simulink model "TFlex_ISSGP_Twin"  (R2018b)
settings: Solver=VariableStepAuto  StartTime=0.0  StopTime=t_end  RelTol=1e-3
values from neighbouring files (symbols this model uses):
  beta_init = 1    [TFlex_ISSGP_Twin_init.m]    (also in TFlex_ISSGP_init.m)
  beta_min = 0.0000    (= 0)    [TFlex_ISSGP_Twin_init.m]    (also in TFlex_ISSGP_init.m)
  beta_reduc = 0.991    [TFlex_ISSGP_Twin_init.m]    (also in TFlex_ISSGP_init.m = nthroot(beta_T/beta_init,(t_hypUpdate(2)-t_hypUpdate(1))/ts_)
  bufferResamp = 50    [TFlex_ISSGP_Twin_init.m]    (also in TFlex_ISSGP_init.m = 10)
  bufferSize = 25    [TFlex_ISSGP_Twin_init.m]    (also in TFlex_ISSGP_init.m = 250)
  D = 80    [TFlex_ISSGP_Twin_init.m]    (also in TFlex_ISSGP_init.m)
  ell = ones(1,n).*0.1    [TFlex_ISSGP_Twin_init.m]    (also in TFlex_ISSGP_init.m = [0.5091   0.0036538   0.0012249])
  ell_init = ell    [TFlex_ISSGP_Twin_init.m]    (also in TFlex_ISSGP_init.m)
  mu_X = [0,0,0]    [TFlex_ISSGP_Twin_init.m]    (also in TFlex_ISSGP_init.m)
  mu_Y = 0    [TFlex_ISSGP_Twin_init.m]    (also in TFlex_ISSGP_init.m)
  n = 3    [TFlex_ISSGP_Twin_init.m]    (also in TFlex_ISSGP_init.m)
  RAND = randn(D,n)    [TFlex_ISSGP_Twin_init.m]    (also in TFlex_ISSGP_init.m)
  RAND2 = randn(D,n)    [TFlex_ISSGP_Twin_init.m]
  sf = 1    [TFlex_ISSGP_Twin_init.m]    (also in TFlex_ISSGP_init.m = 111.9926)
  sf_init = sf    (= 1)    [TFlex_ISSGP_Twin_init.m]    (also in TFlex_ISSGP_init.m = 111.9926)
  sig_X = [1,1,1]    [TFlex_ISSGP_Twin_init.m]    (also in TFlex_ISSGP_init.m)
  sig_Y = 1    [TFlex_ISSGP_Twin_init.m]    (also in TFlex_ISSGP_init.m)
  SIGMA2_init = RAND2.*ell    [TFlex_ISSGP_Twin_init.m]
  SIGMA_init = RAND.*ell    [TFlex_ISSGP_Twin_init.m]    (also in TFlex_ISSGP_init.m)
  sn = 2.303584    [TFlex_ISSGP_Twin_init.m]    (also in TFlex_ISSGP_init.m)
  sn2 = sn    (= 2.303584)    [TFlex_ISSGP_Twin_init.m]
  t_hypUpdate = [10 55]    [TFlex_ISSGP_Twin_init.m]    (also in TFlex_ISSGP_init.m = [t_end t_end+1])
  t_hypUpdate2 = [70 115]    [TFlex_ISSGP_Twin_init.m]
  t_learn = 55    [TFlex_ISSGP_Twin_init.m]    (also in TFlex_ISSGP_init.m = 5)
  t_learn2 = 115    [TFlex_ISSGP_Twin_init.m]
  t_predict = 65    [TFlex_ISSGP_Twin_init.m]    (also in TFlex_ISSGP_init.m = 15)
  t_predict2 = 125    [TFlex_ISSGP_Twin_init.m]
  ts = 1/1000    (= 0.001)    [TFlex_ISSGP_Twin_init.m]    (also in TFlex_ISSGP_init.m)
  ts_opti = ts*100    (= 0.1)    [TFlex_ISSGP_Twin_init.m]    (also in TFlex_ISSGP_init.m)
  Z = bufferSize*bufferResamp    (= 1250)    [TFlex_ISSGP_Twin_init.m]    (also in TFlex_ISSGP_init.m = 2500)
undefined symbols (not defined in the file or in its folder): Cogging, DiscIntNeverNeededParam, I_limit, PID, Plant, R1, R2, Reference, SVF, X, Y
libraries: simulink x6
settings Model: Creator=wout7  LastModifiedBy=wout7

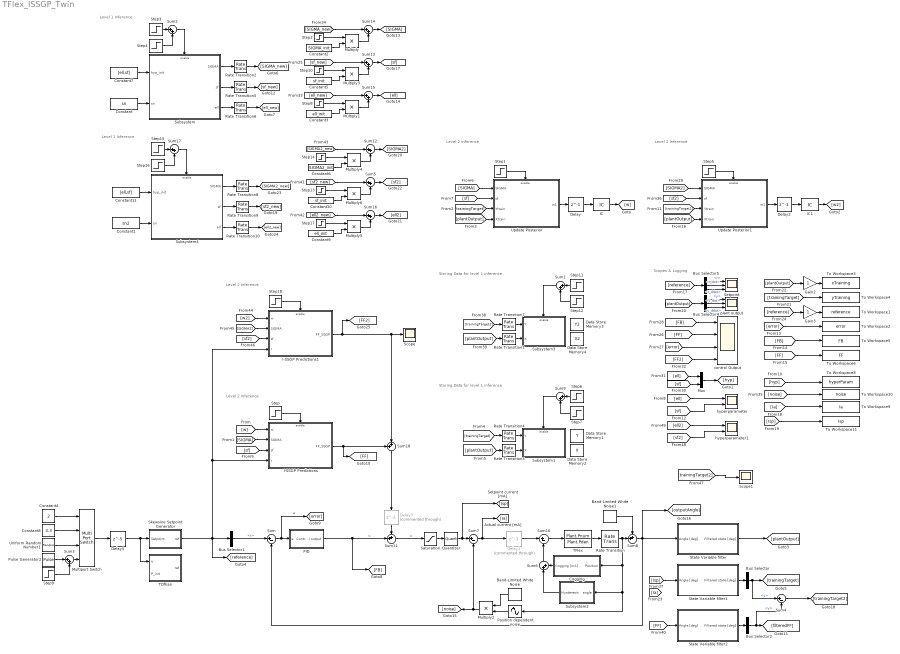
== system TFlex_ISSGP_Twin ==
  note: Storing Data for level 1 inference
  note: Scopes & Logging
  note: Level 1 Inference
  note: Level 2 Inference
  note: Level 2 Inference
  note: Level 2 Inference
  note: Storing Data for level 1 inference
  note: Level 1 Inference
  note: Level 2 Inference
  Band-Limited White Noise : simulink/Sources/Band-Limited White Noise  Cov=[1e-9]  Ts=ts  seed=48124
  Band-Limited White Noise1 : simulink/Sources/Band-Limited White Noise  Cov=[1e-15]  Ts=ts  seed=[23341]
  Bus Selector : BusSelector  OutputSignals=y
  Bus Selector1 : BusSelector  OutputSignals=r
  Bus Selector2 : BusSelector  OutputSignals=y
  Bus Selector4 : BusSelector  OutputSignals=y,y_dot,y_ddot
  Bus Selector5 : BusSelector  OutputSignals=r,r_dot,r_ddot
  Cogging : Subsystem
  Constant : Constant  Value=sn  SampleTime=ts_opti
  Constant1 : Constant  Value=sn2  SampleTime=ts_opti
  Constant10 : Constant  Value=sf_init  SampleTime=ts_opti
  Constant11 : Constant  Value=[ell,sf]  VectorParams1D=off  SampleTime=ts_opti
  Constant2 : Constant  Value=SIGMA_init  SampleTime=ts_opti
  Constant3 : Constant  Value=ell_init  SampleTime=ts_opti
  Constant4 : Constant  Value=2  SampleTime=Reference.ts
  Constant5 : Constant  Value=sf_init  SampleTime=ts_opti
  Constant6 : Constant  Value=SIGMA2_init  SampleTime=ts_opti
  Constant7 : Constant  Value=[ell,sf]  VectorParams1D=off  SampleTime=ts_opti
  Constant8 : Constant  Value=3.3  SampleTime=Reference.ts
  Constant9 : Constant  Value=ell_init  SampleTime=ts_opti
  Data Store Memory1 : DataStoreMemory  DataStoreName=Y  ReadBeforeWriteMsg=warning  WriteAfterWriteMsg=warning  WriteAfterReadMsg=warning  InitialValue=zeros(bufferSize,1)  VectorParams1D=off  ShowAdditionalParam=off  OutDataTypeStr=double
      settings: LockScale=on
  Data Store Memory2 : DataStoreMemory  DataStoreName=X  ReadBeforeWriteMsg=warning  WriteAfterWriteMsg=warning  WriteAfterReadMsg=warning  InitialValue=zeros(bufferSize,3)  VectorParams1D=off  ShowAdditionalParam=off  OutDataTypeStr=double
      settings: LockScale=on
  Data Store Memory3 : DataStoreMemory  DataStoreName=Y2  ReadBeforeWriteMsg=warning  WriteAfterWriteMsg=warning  WriteAfterReadMsg=warning  InitialValue=zeros(bufferSize,1)  VectorParams1D=off  ShowAdditionalParam=off  OutDataTypeStr=double
      settings: LockScale=on
  Data Store Memory4 : DataStoreMemory  DataStoreName=X2  ReadBeforeWriteMsg=warning  WriteAfterWriteMsg=warning  WriteAfterReadMsg=warning  InitialValue=zeros(bufferSize,3)  VectorParams1D=off  ShowAdditionalParam=off  OutDataTypeStr=double
      settings: LockScale=on
  Delay : Delay  DelayLength=1  InitialCondition=0
  Delay1 : Delay  Commented=through  DelayLength=3  InitialCondition=0
  Delay2 : Delay  DelayLength=1  InitialCondition=0
  Delay3 : Delay  Commented=through  DelayLength=3  InitialCondition=0
  Delay5 : Delay  DelayLength=5  SampleTime=Reference.ts
  Gain2 : Gain
  Gain3 : Gain
  I-SSGP Predictions : Subsystem
  I-SSGP Predictions1 : Subsystem
  IC : InitialCondition  Value=ones(2*D,1)*0.001
  IC1 : InitialCondition  Value=ones(2*D,1)*0.001
  Multiply{,1..6} (7 alike) : Product
  Multiport Switch : MultiPortSwitch
  Mux : Mux  Inputs=2
  PID : Subsystem
  Position dependent noise : Sin  TimeSource=Use external signal  Amplitude=2.5  Bias=7.4979  Frequency=2*pi/13  SampleTime=0
  Pulse Generator2 : DiscretePulseGenerator  Amplitude=2*24  SampleTime=Reference.ts
  Quantizer : Quantizer  QuantizationInterval=1
  Rate Transition{,2,5..6,8..10} (7 alike) : RateTransition  OutPortSampleTime=ts
  Rate Transition1 : RateTransition  OutPortSampleTime=ts*10
  Rate Transition3 : RateTransition  OutPortSampleTime=ts*bufferResamp
  Rate Transition4 : RateTransition  OutPortSampleTime=ts*bufferResamp
  Rate Transition7 : RateTransition  OutPortSampleTime=ts*10
  Saturation : Saturate  UpperLimit=I_limit  LowerLimit=-I_limit
  Scope : Scope
  Scope1 : Scope
  Setpoint : Scope  NumInputPorts=3
  Skewsine Setpoint Generator : Subsystem
  State Variable filter : Subsystem
  State Variable filter1 : Subsystem
  State Variable filter2 : Subsystem
  Step : Step  Time=t_predict  SampleTime=ts
  Step1 : Step  Time=t_learn  SampleTime=ts
  Step{2,8,10,13..14,17} (6 alike) : Step  Time=t_hypUpdate(1)+ts  Before=1  After=0  SampleTime=ts_opti
  Step11 : Step  Time=t_hypUpdate2(2)  After=-1  SampleTime=ts_opti
  Step12 : Step  Time=t_hypUpdate2(1)-Z*ts  SampleTime=ts_opti
  Step15 : Step  Time=t_hypUpdate2(2)  After=-1  SampleTime=ts_opti
  Step16 : Step  Time=t_hypUpdate2(1)  SampleTime=ts_opti
  Step18 : Step  Time=t_predict2  SampleTime=ts
  Step3 : Step  Time=t_hypUpdate(2)  After=-1  SampleTime=ts_opti
  Step4 : Step  Time=t_hypUpdate(1)  SampleTime=ts_opti
  Step5 : Step  Time=t_learn2  SampleTime=ts
  Step6 : Step  Time=t_hypUpdate(2)  After=-1  SampleTime=ts_opti
  Step7 : Step  Time=t_hypUpdate(1)-Z*ts  SampleTime=ts_opti
  Step9 : Step  Time=0  After=-24  SampleTime=Reference.ts
  Subsystem : Subsystem
  Subsystem1 : Subsystem
  Subsystem2 : Subsystem
  Subsystem3 : Subsystem
  Subsystem4 : Subsystem
  Sum{,4,7,10} (4 alike) : Sum  Inputs=|+-
  Sum{1..3,5..6,9,12..17} (12 alike) : Sum  Inputs=|++
  Sum11 : Sum  Inputs=++|
  Sum18 : Sum  Inputs=++|
  Sum8 : Sum  Inputs=++|
  TDfhan : Subsystem
  TFlex : TransferFcn  Numerator=Plant.Pnum  Denominator=Plant.Pden  ContinuousStateAttributes='angle'
  To Workspace1 : ToWorkspace  VariableName=reference  SampleTime=-1
  To Workspace10 : ToWorkspace  VariableName=noise  SampleTime=-1
  To Workspace11 : ToWorkspace  VariableName=Isp  SampleTime=-1
  To Workspace2 : ToWorkspace  VariableName=error  SampleTime=-1
  To Workspace3 : ToWorkspace  VariableName=xTraining  SampleTime=-1
  To Workspace4 : ToWorkspace  VariableName=yTraining  SampleTime=-1
  To Workspace5 : ToWorkspace  VariableName=FB  SampleTime=-1
  To Workspace6 : ToWorkspace  VariableName=FF  SampleTime=-1
  To Workspace8 : ToWorkspace  VariableName=hyperParam  SampleTime=-1
  To Workspace9 : ToWorkspace  VariableName=Ia  SampleTime=-1
  Uniform Random Number1 : UniformRandomNumber  Minimum=-23  Maximum=23  Seed=Reference.seed  SampleTime=Reference.ts
  Update Posterior : Subsystem
  Update Posterior1 : Subsystem
  control Output : Scope  NumInputPorts=4
  hyperparameter : Scope  NumInputPorts=2
  hyperparameter1 : Scope  NumInputPorts=2
  plant output : Scope  NumInputPorts=3
  wires:
  Sum/1 -> PID/1(e), [error]  "e"
  Sum8/1 -> State Variable filter/1(Angle [deg]), [outputAngle], Sum/2
  Bus Selector1/1 -> Sum/1  "<r>"
  Update Posterior/1(w1) -> Delay/1
  Step/1 -> I-SSGP Predictions/Enable
  Step1/1 -> Update Posterior/Enable
  IC/1 -> [w]
  [w] -> I-SSGP Predictions/1(w)
  [sf] -> Update Posterior/2(sf)
  [SIGMA] -> I-SSGP Predictions/2(SIGMA)
  Delay/1 -> IC/1
  [trainingTarget] -> Update Posterior/3(Ytrain)
  [SIGMA] -> Update Posterior/1(SIGMA)
  Constant7/1 -> Subsystem/1(hyp_init)
  Step4/1 -> Sum2/2
  Step3/1 -> Sum2/1
  Sum2/1 -> Subsystem/Enable
  [sf] -> I-SSGP Predictions/3(sf)
  TFlex/1 -> Rate Transition/1
  [reference] -> Gain3/1
  Bus Selector5/2 -> Setpoint/2  "<r_dot>"
  Bus Selector5/1 -> Setpoint/1  "<r>"
  [error] -> To Workspace2/1
  Bus Selector5/3 -> Setpoint/3  "<r_ddot>"
  [FB] -> To Workspace5/1
  [plantOutput] -> Gain2/1
  Gain2/1 -> To Workspace3/1
  [plantOutput] -> Bus Selector4/1
  Gain3/1 -> To Workspace1/1
  Bus Selector4/1 -> plant output/1  "<y>"
  Bus Selector4/3 -> plant output/3  "<y_ddot>"
  [reference] -> Bus Selector5/1
  [trainingTarget] -> To Workspace4/1
  Bus Selector4/2 -> plant output/2  "<y_dot>"
  [FF] -> To Workspace6/1
  [FF] -> control Output/2
  [error] -> control Output/3
  [FB] -> control Output/1
  Step7/1 -> Sum9/2
  Sum9/1 -> Subsystem1/Enable
  Step6/1 -> Sum9/1
  Subsystem/2(sf) -> Rate Transition5/1
  Subsystem/1(SIGMA) -> Rate Transition2/1
  Subsystem/3(ell) -> Rate Transition6/1
  [ell] -> hyperparameter/1
  [hyp] -> To Workspace8/1
  [sf] -> hyperparameter/2
  [sf] -> Mux/2
  [ell] -> Mux/1
  Mux/1 -> [hyp]
  [plantOutput] -> Rate Transition3/1
  Rate Transition3/1 -> Subsystem1/2(X)
  [trainingTarget] -> Rate Transition4/1
  Rate Transition4/1 -> Subsystem1/1(Y)
  Rate Transition2/1 -> [SIGMA_new]
  Rate Transition5/1 -> [sf_new]
  Rate Transition6/1 -> [ell_new]
  [SIGMA_new] -> Sum14/1
  Step2/1 -> Multiply/1
  Constant2/1 -> Multiply/2
  Multiply/1 -> Sum14/2
  Sum14/1 -> [SIGMA]
  [plantOutput] -> Update Posterior/4(Xtrain)
  Saturation/1 -> Quantizer/1
  PID/1(Control output) -> [FB], Sum11/2  "u"
  State Variable filter/1(Filtered state [deg]) -> [plantOutput]
  Rate Transition/1 -> Sum8/2, Cogging/1(Position), Subsystem2/1(angle), Position dependent noise/1
  Sum11/1 -> Saturation/1  "u"
  Sum10/1 -> TFlex/1
  State Variable filter1/1(Filtered state [deg]) -> Bus Selector/1
  Sum7/1 -> Delay1/1, [Ia]
  Multiply2/1 -> Sum7/2, [noise]
  [sf_new] -> Sum13/1
  Step10/1 -> Multiply3/1
  Multiply3/1 -> Sum13/2
  Sum13/1 -> [sf]
  Constant5/1 -> Multiply3/2
  [ell_new] -> Sum15/1
  Step8/1 -> Multiply1/1
  Multiply1/1 -> Sum15/2
  Sum15/1 -> [ell]
  Constant3/1 -> Multiply1/2
  Cogging/1(Cogging [mA]) -> Sum6/2
  Quantizer/1 -> [Isp], Sum7/1
  I-SSGP Predictions/1(FF_SSGP) -> [FF], Sum18/1
  Delay3/1 -> Sum11/1
  Band-Limited White Noise/1 -> Multiply2/1
  Position dependent noise/1 -> Multiply2/2
  Constant/1 -> Subsystem/2(sn)
  [noise] -> To Workspace10/1
  Pulse Generator2/1 -> Sum3/1
  Sum3/1 -> Multiport Switch/4
  Step9/1 -> Sum3/2
  Constant4/1 -> Multiport Switch/1
  Uniform Random Number1/1 -> Multiport Switch/3
  Constant8/1 -> Multiport Switch/2
  [Ia] -> To Workspace9/1
  [Isp] -> To Workspace11/1
  Band-Limited White Noise1/1 -> Sum8/1
  Delay1/1 -> Sum10/1
  [Isp] -> State Variable filter1/1(Angle [deg])
  Bus Selector/1 -> Sum4/1, [trainingTarget]  "<y>"
  Sum6/1 -> Sum10/2
  Multiport Switch/1 -> Delay5/1
  Delay5/1 -> Skewsine Setpoint Generator/1(Setpoint), TDfhan/1(V)
  Subsystem2/1(Hysteresis) -> Sum6/1
  Update Posterior1/1(w1) -> Delay2/1
  [plantOutput] -> Update Posterior1/4(Xtrain)
  IC1/1 -> [w2]
  [trainingTarget2] -> Update Posterior1/3(Ytrain)
  [sf2] -> Update Posterior1/2(sf)
  Step5/1 -> Update Posterior1/Enable
  [SIGMA2] -> Update Posterior1/1(SIGMA)
  Delay2/1 -> IC1/1
  Sum1/1 -> Subsystem3/Enable
  Step11/1 -> Sum1/1
  [plantOutput] -> Rate Transition1/1
  [trainingTarget2] -> Rate Transition7/1
  Rate Transition1/1 -> Subsystem3/2(X)
  Step12/1 -> Sum1/2
  Rate Transition7/1 -> Subsystem3/1(Y)
  [FF] -> State Variable filter2/1(Angle [deg])
  State Variable filter2/1(Filtered state [deg]) -> Bus Selector2/1
  Bus Selector2/1 -> Sum4/2, [filteredFF]  "<y>"
  Sum4/1 -> [trainingTarget2]
  Sum12/1 -> [SIGMA2]
  Rate Transition9/1 -> [sf2_new]
  Sum5/1 -> [sf2]
  Constant10/1 -> Multiply6/2
  Sum16/1 -> [ell2]
  Step17/1 -> Multiply5/1
  Step13/1 -> Multiply6/1
  [ell2_new] -> Sum16/1
  Constant9/1 -> Multiply5/2
  Step15/1 -> Sum17/1
  Multiply5/1 -> Sum16/2
  Multiply6/1 -> Sum5/2
  [SIGMA2_new] -> Sum12/1
  Rate Transition10/1 -> [ell2_new]
  Rate Transition8/1 -> [SIGMA2_new]
  Constant6/1 -> Multiply4/2
  Constant1/1 -> Subsystem4/2(sn)
  Subsystem4/1(SIGMA) -> Rate Transition8/1
  Subsystem4/3(ell) -> Rate Transition10/1
  Multiply4/1 -> Sum12/2
  Constant11/1 -> Subsystem4/1(hyp_init)
  Subsystem4/2(sf) -> Rate Transition9/1
  [sf2_new] -> Sum5/1
  Sum17/1 -> Subsystem4/Enable
  Step16/1 -> Sum17/2
  Step14/1 -> Multiply4/1
  [w2] -> I-SSGP Predictions1/1(w)
  Step18/1 -> I-SSGP Predictions1/Enable
  Skewsine Setpoint Generator/1(ref) -> I-SSGP Predictions1/4(r), I-SSGP Predictions/4(r), [reference], Bus Selector1/1
  [sf2] -> I-SSGP Predictions1/3(sf)
  [SIGMA2] -> I-SSGP Predictions1/2(SIGMA)
  Sum18/1 -> Delay3/1
  I-SSGP Predictions1/1(FF_SSGP) -> [FF2], Sum18/2, Scope/1
  [trainingTarget2] -> Scope1/1
  [ell2] -> hyperparameter1/1
  [sf2] -> hyperparameter1/2
  [FF2] -> control Output/4

== system TFlex_ISSGP_Twin/Cogging ==
  Position : Inport
  Gain : Gain  Gain=20
  Scope : Scope
  Sine Wave Function : Sin  TimeSource=Use external signal  Amplitude=Cogging.amplitude  Frequency=2*pi./Cogging.frequency  Phase=Cogging.phase*2*pi  SampleTime=0
  Sum of Elements : Sum  Inputs=+
  Cogging [mA] : Outport
  wires:
  Gain/1 -> Scope/1, [Cogging], Cogging [mA]/1
  Sum of Elements/1 -> Gain/1
  Position/1 -> Sine Wave Function/1
  Sine Wave Function/1 -> Sum of Elements/1

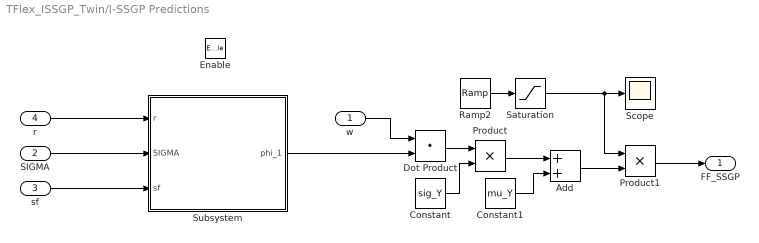
== system TFlex_ISSGP_Twin/I-SSGP Predictions ==
  w : Inport
  SIGMA : Inport  Port=2
  sf : Inport  Port=3
  r : Inport  Port=4
  Enable : EnablePort
  Add : Sum
  Constant : Constant  Value=sig_Y  VectorParams1D=off  SampleTime=ts
  Constant1 : Constant  Value=mu_Y  VectorParams1D=off  SampleTime=ts
  Dot Product : DotProduct  OutDataTypeStr=Inherit: Inherit via internal rule
  Product : Product
  Product1 : Product
  Ramp2 : simulink/Sources/Ramp  slope=1/10  start=t_predict  InitialOutput=0
  Saturation : Saturate  UpperLimit=1  LowerLimit=0
  Scope : Scope
  Subsystem : Subsystem
  FF_SSGP : Outport  SampleTime=ts
  wires:
  w/1 -> Dot Product/1
  Subsystem/1(phi_1) -> Dot Product/2
  SIGMA/1 -> Subsystem/2(SIGMA)
  Dot Product/1 -> Product/1
  Constant/1 -> Product/2
  Product/1 -> Add/1
  Constant1/1 -> Add/2
  Product1/1 -> FF_SSGP/1
  Ramp2/1 -> Saturation/1
  Add/1 -> Product1/2
  sf/1 -> Subsystem/3(sf)
  Saturation/1 -> Product1/1, Scope/1
  r/1 -> Subsystem/1(r)

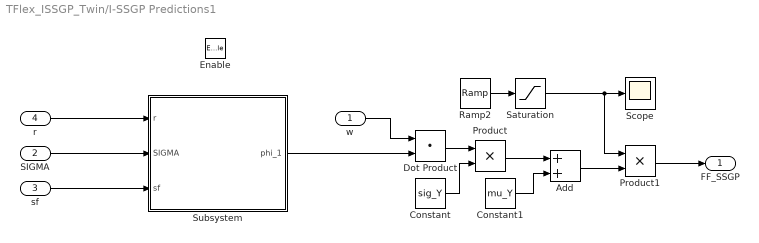
== system TFlex_ISSGP_Twin/I-SSGP Predictions1 ==
  w : Inport
  SIGMA : Inport  Port=2
  sf : Inport  Port=3
  r : Inport  Port=4
  Enable : EnablePort
  Add : Sum
  Constant : Constant  Value=sig_Y  VectorParams1D=off  SampleTime=ts
  Constant1 : Constant  Value=mu_Y  VectorParams1D=off  SampleTime=ts
  Dot Product : DotProduct  OutDataTypeStr=Inherit: Inherit via internal rule
  Product : Product
  Product1 : Product
  Ramp2 : simulink/Sources/Ramp  slope=1/10  start=t_predict  InitialOutput=0
  Saturation : Saturate  UpperLimit=1  LowerLimit=0
  Scope : Scope
  Subsystem : Subsystem
  FF_SSGP : Outport  SampleTime=ts
  wires:
  w/1 -> Dot Product/1
  Subsystem/1(phi_1) -> Dot Product/2
  SIGMA/1 -> Subsystem/2(SIGMA)
  Dot Product/1 -> Product/1
  Constant/1 -> Product/2
  Product/1 -> Add/1
  Constant1/1 -> Add/2
  Product1/1 -> FF_SSGP/1
  Ramp2/1 -> Saturation/1
  Add/1 -> Product1/2
  sf/1 -> Subsystem/3(sf)
  Saturation/1 -> Product1/1, Scope/1
  r/1 -> Subsystem/1(r)

== system TFlex_ISSGP_Twin/PID ==
  e : Inport
  Discrete Derivative : simulink/Discrete/Discrete Derivative  gainval=1.0  ICPrevScaledInput=0.0  OutMin=[]  OutMax=[]  OutDataType=fixdt(1, 16)  OutScaling=2^-10  DoSatur=off
  Discrete-Time Integrator2 : DiscreteIntegrator  SampleTime=-1  ICPrevOutput=DiscIntNeverNeededParam  ICPrevScaledInput=DiscIntNeverNeededParam
  Gain1 : Gain  Gain=PID.Kp
  Gain2 : Gain  Gain=PID.Ki
  Gain3 : Gain  Gain=PID.Kd
  Lowpass : DiscreteTransferFcn  Numerator=PID.LPnum  Denominator=PID.LPden  SampleTime=ts
  Sum2 : Sum  Inputs=3
  Control output : Outport
  wires:
  Discrete-Time Integrator2/1 -> Gain2/1
  Gain1/1 -> Sum2/2
  Gain2/1 -> Sum2/1
  Gain3/1 -> Sum2/3
  Sum2/1 -> Control output/1
  e/1 -> Discrete-Time Integrator2/1, Gain1/1, Lowpass/1
  Lowpass/1 -> Discrete Derivative/1
  Discrete Derivative/1 -> Gain3/1

== system TFlex_ISSGP_Twin/Skewsine Setpoint Generator ==
  Setpoint : Inport
  Bus Creator : BusCreator  Inputs=3
  Subsystem : Subsystem
  ref : Outport
  wires:
  Subsystem/3(r_ddot) -> Bus Creator/3  "r_ddot"
  Bus Creator/1 -> ref/1
  Subsystem/2(r_dot) -> Bus Creator/2  "r_dot"
  Subsystem/1(r) -> Bus Creator/1  "r"
  Setpoint/1 -> Subsystem/1(setpoint)

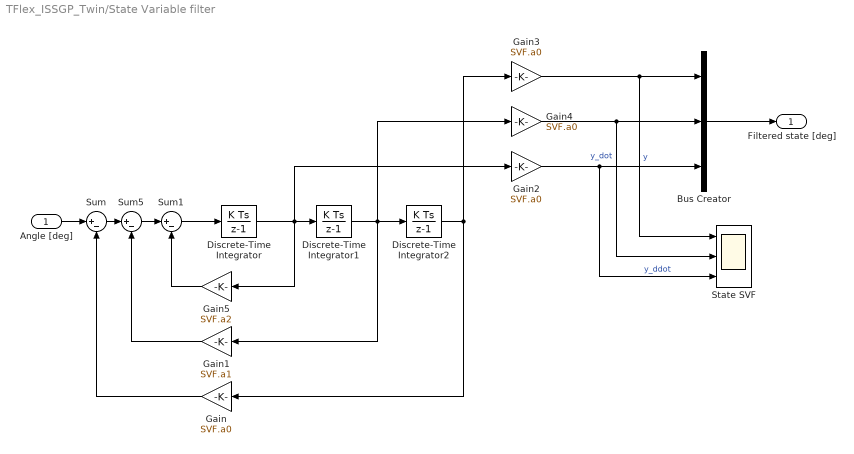
== system TFlex_ISSGP_Twin/State Variable filter ==
  Angle [deg] : Inport
  Bus Creator : BusCreator  Inputs=3
  Discrete-Time Integrator : DiscreteIntegrator  SampleTime=-1  ICPrevOutput=DiscIntNeverNeededParam  ICPrevScaledInput=DiscIntNeverNeededParam
  Discrete-Time Integrator1 : DiscreteIntegrator  SampleTime=-1  ICPrevOutput=DiscIntNeverNeededParam  ICPrevScaledInput=DiscIntNeverNeededParam
  Discrete-Time Integrator2 : DiscreteIntegrator  SampleTime=-1  ICPrevOutput=DiscIntNeverNeededParam  ICPrevScaledInput=DiscIntNeverNeededParam
  Gain{,2..4} (4 alike) : Gain  Gain=SVF.a0
  Gain1 : Gain  Gain=SVF.a1
  Gain5 : Gain  Gain=SVF.a2
  State SVF : Scope  NumInputPorts=3
  Sum : Sum  Inputs=|+-
  Sum1 : Sum  Inputs=|+-
  Sum5 : Sum  Inputs=|+-
  Filtered state [deg] : Outport  SampleTime=ts
  wires:
  Bus Creator/1 -> Filtered state [deg]/1
  Sum1/1 -> Discrete-Time Integrator/1
  Angle [deg]/1 -> Sum/1
  Sum/1 -> Sum5/1
  Gain/1 -> Sum/2
  Gain1/1 -> Sum5/2
  Gain3/1 -> State SVF/1, Bus Creator/1  "y"
  Gain2/1 -> State SVF/3, Bus Creator/3  "y_ddot"
  Gain4/1 -> State SVF/2, Bus Creator/2  "y_dot"
  Gain5/1 -> Sum1/2
  Sum5/1 -> Sum1/1
  Discrete-Time Integrator/1 -> Discrete-Time Integrator1/1, Gain2/1, Gain5/1
  Discrete-Time Integrator1/1 -> Discrete-Time Integrator2/1, Gain4/1, Gain1/1
  Discrete-Time Integrator2/1 -> Gain3/1, Gain/1

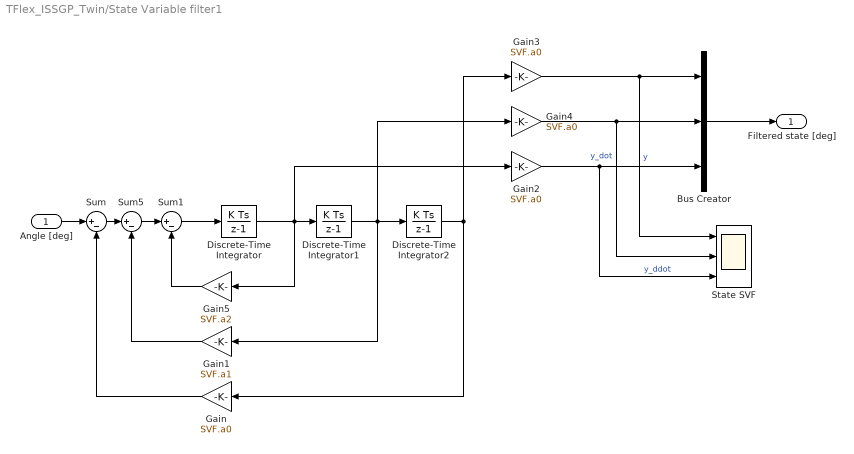
== system TFlex_ISSGP_Twin/State Variable filter1 ==
  Angle [deg] : Inport
  Bus Creator : BusCreator  Inputs=3
  Discrete-Time Integrator : DiscreteIntegrator  SampleTime=-1  ICPrevOutput=DiscIntNeverNeededParam  ICPrevScaledInput=DiscIntNeverNeededParam
  Discrete-Time Integrator1 : DiscreteIntegrator  SampleTime=-1  ICPrevOutput=DiscIntNeverNeededParam  ICPrevScaledInput=DiscIntNeverNeededParam
  Discrete-Time Integrator2 : DiscreteIntegrator  SampleTime=-1  ICPrevOutput=DiscIntNeverNeededParam  ICPrevScaledInput=DiscIntNeverNeededParam
  Gain{,2..4} (4 alike) : Gain  Gain=SVF.a0
  Gain1 : Gain  Gain=SVF.a1
  Gain5 : Gain  Gain=SVF.a2
  State SVF : Scope  NumInputPorts=3
  Sum : Sum  Inputs=|+-
  Sum1 : Sum  Inputs=|+-
  Sum5 : Sum  Inputs=|+-
  Filtered state [deg] : Outport  SampleTime=ts
  wires:
  Bus Creator/1 -> Filtered state [deg]/1
  Sum1/1 -> Discrete-Time Integrator/1
  Angle [deg]/1 -> Sum/1
  Sum/1 -> Sum5/1
  Gain/1 -> Sum/2
  Gain1/1 -> Sum5/2
  Gain3/1 -> State SVF/1, Bus Creator/1  "y"
  Gain2/1 -> State SVF/3, Bus Creator/3  "y_ddot"
  Gain4/1 -> State SVF/2, Bus Creator/2  "y_dot"
  Gain5/1 -> Sum1/2
  Sum5/1 -> Sum1/1
  Discrete-Time Integrator/1 -> Discrete-Time Integrator1/1, Gain2/1, Gain5/1
  Discrete-Time Integrator1/1 -> Discrete-Time Integrator2/1, Gain4/1, Gain1/1
  Discrete-Time Integrator2/1 -> Gain3/1, Gain/1

== system TFlex_ISSGP_Twin/State Variable filter2 ==
  Angle [deg] : Inport
  Bus Creator : BusCreator  Inputs=3
  Discrete-Time Integrator : DiscreteIntegrator  SampleTime=-1  ICPrevOutput=DiscIntNeverNeededParam  ICPrevScaledInput=DiscIntNeverNeededParam
  Discrete-Time Integrator1 : DiscreteIntegrator  SampleTime=-1  ICPrevOutput=DiscIntNeverNeededParam  ICPrevScaledInput=DiscIntNeverNeededParam
  Discrete-Time Integrator2 : DiscreteIntegrator  SampleTime=-1  ICPrevOutput=DiscIntNeverNeededParam  ICPrevScaledInput=DiscIntNeverNeededParam
  Gain{,2..4} (4 alike) : Gain  Gain=SVF.a0
  Gain1 : Gain  Gain=SVF.a1
  Gain5 : Gain  Gain=SVF.a2
  State SVF : Scope  NumInputPorts=3
  Sum : Sum  Inputs=|+-
  Sum1 : Sum  Inputs=|+-
  Sum5 : Sum  Inputs=|+-
  Filtered state [deg] : Outport  SampleTime=ts
  wires:
  Bus Creator/1 -> Filtered state [deg]/1
  Sum1/1 -> Discrete-Time Integrator/1
  Angle [deg]/1 -> Sum/1
  Sum/1 -> Sum5/1
  Gain/1 -> Sum/2
  Gain1/1 -> Sum5/2
  Gain3/1 -> State SVF/1, Bus Creator/1  "y"
  Gain2/1 -> State SVF/3, Bus Creator/3  "y_ddot"
  Gain4/1 -> State SVF/2, Bus Creator/2  "y_dot"
  Gain5/1 -> Sum1/2
  Sum5/1 -> Sum1/1
  Discrete-Time Integrator/1 -> Discrete-Time Integrator1/1, Gain2/1, Gain5/1
  Discrete-Time Integrator1/1 -> Discrete-Time Integrator2/1, Gain4/1, Gain1/1
  Discrete-Time Integrator2/1 -> Gain3/1, Gain/1

== system TFlex_ISSGP_Twin/Subsystem ==
  hyp_init : Inport  PortDimensions=[1,n+1]
  sn : Inport  Port=2
  Enable : EnablePort
  Bus Creator : BusCreator  Inputs=3
  Constant13 : Constant  Value=RAND  VectorParams1D=off  SampleTime=ts_opti
  Data Store Read : DataStoreRead  DataStoreName=Y  SampleTime=ts_opti  DataStoreElements=Y(:,:)
  Data Store Read1 : DataStoreRead  DataStoreName=X  SampleTime=ts_opti  DataStoreElements=X(:,:)
  Demux : Demux
  MATLAB Function : MATLAB Function  TreatAsAtomicUnit=on
  MATLAB Function1 : MATLAB Function  TreatAsAtomicUnit=on
  Scope : Scope
  SIGMA : Outport
  sf : Outport  Port=2
  ell : Outport  Port=3
  wires:
  hyp_init/1 -> MATLAB Function/1(hyp_init)
  MATLAB Function/2(beta_out) -> Scope/1  "beta"
  Data Store Read1/1 -> MATLAB Function/2(x)
  Data Store Read/1 -> MATLAB Function/3(y)
  sn/1 -> MATLAB Function/4(sn2)
  Demux/4 -> sf/1  "sf"
  Constant13/1 -> MATLAB Function1/1(RAND)
  MATLAB Function1/1(SIGMA) -> SIGMA/1
  MATLAB Function/1(hyp_opt) -> Demux/1, MATLAB Function1/2(hyp)
  Demux/1 -> Bus Creator/1  "l_1"
  Demux/2 -> Bus Creator/2  "l_2"
  Demux/3 -> Bus Creator/3  "l_3"
  Bus Creator/1 -> ell/1

== system TFlex_ISSGP_Twin/Subsystem1 ==
  Y : Inport
  X : Inport  Port=2
  Enable : EnablePort
  Add1 : Sum  Inputs=+-
  Add2 : Sum  Inputs=+-
  Bus Selector : BusSelector  OutputSignals=y,y_dot,y_ddot
  Constant3 : Constant  Value=sig_X  VectorParams1D=off  SampleTime=ts_opti
  Constant4 : Constant  Value=mu_X  VectorParams1D=off  SampleTime=ts_opti
  Constant8 : Constant  Value=sig_Y  VectorParams1D=off  SampleTime=ts_opti
  Constant9 : Constant  Value=mu_Y  VectorParams1D=off  SampleTime=ts_opti
  Divide : Product  Inputs=*/
  Divide1 : Product  Inputs=*/
  MATLAB Function1 : MATLAB Function  TreatAsAtomicUnit=on
  MATLAB Function2 : MATLAB Function  TreatAsAtomicUnit=on
  Scope : Scope  NumInputPorts=3
  wires:
  Divide1/1 -> MATLAB Function2/1(x)
  Y/1 -> Add1/1
  Divide/1 -> MATLAB Function1/1(y)
  Add1/1 -> Divide/1
  Add2/1 -> Divide1/1
  Constant9/1 -> Add1/2
  Constant3/1 -> Divide1/2
  Constant4/1 -> Add2/2
  Constant8/1 -> Divide/2
  Bus Selector/1 -> Scope/1  "<y>"
  Bus Selector/2 -> Scope/2  "<y_dot>"
  Bus Selector/3 -> Scope/3  "<y_ddot>"
  X/1 -> Add2/1, Bus Selector/1

== system TFlex_ISSGP_Twin/Subsystem2 ==
  angle : Inport
  Discrete Derivative : simulink/Discrete/Discrete Derivative  gainval=1.0  ICPrevScaledInput=0.0  OutMin=[]  OutMax=[]  OutDataType=fixdt(1, 16)  OutScaling=2^-10  DoSatur=off
  Discrete-Time Integrator : DiscreteIntegrator  SampleTime=-1  ICPrevOutput=DiscIntNeverNeededParam  ICPrevScaledInput=DiscIntNeverNeededParam
  MATLAB Function : MATLAB Function  TreatAsAtomicUnit=on
  Sum1 : Sum  Inputs=|+-
  Hysteresis : Outport
  wires:
  MATLAB Function/1(y) -> Sum1/2
  angle/1 -> Discrete Derivative/1
  Sum1/1 -> Discrete-Time Integrator/1
  Discrete Derivative/1 -> Sum1/1, MATLAB Function/1(Vr)
  Discrete-Time Integrator/1 -> Hysteresis/1, MATLAB Function/2(p)

== system TFlex_ISSGP_Twin/Subsystem3 ==
  Y : Inport
  X : Inport  Port=2
  Enable : EnablePort
  Add1 : Sum  Inputs=+-
  Add2 : Sum  Inputs=+-
  Bus Selector : BusSelector  OutputSignals=y,y_dot,y_ddot
  Constant3 : Constant  Value=sig_X  VectorParams1D=off  SampleTime=ts_opti
  Constant4 : Constant  Value=mu_X  VectorParams1D=off  SampleTime=ts_opti
  Constant8 : Constant  Value=sig_Y  VectorParams1D=off  SampleTime=ts_opti
  Constant9 : Constant  Value=mu_Y  VectorParams1D=off  SampleTime=ts_opti
  Divide : Product  Inputs=*/
  Divide1 : Product  Inputs=*/
  MATLAB Function1 : MATLAB Function  TreatAsAtomicUnit=on
  MATLAB Function2 : MATLAB Function  TreatAsAtomicUnit=on
  Scope : Scope  NumInputPorts=4
  wires:
  Divide1/1 -> MATLAB Function2/1(x)
  Y/1 -> Scope/1, Add1/1
  Divide/1 -> MATLAB Function1/1(y)
  Add1/1 -> Divide/1
  Add2/1 -> Divide1/1
  Constant9/1 -> Add1/2
  Constant3/1 -> Divide1/2
  Constant4/1 -> Add2/2
  Constant8/1 -> Divide/2
  Bus Selector/1 -> Scope/2  "<y>"
  Bus Selector/2 -> Scope/3  "<y_dot>"
  Bus Selector/3 -> Scope/4  "<y_ddot>"
  X/1 -> Add2/1, Bus Selector/1

== system TFlex_ISSGP_Twin/Subsystem4 ==
  hyp_init : Inport  PortDimensions=[1,n+1]
  sn : Inport  Port=2
  Enable : EnablePort
  Bus Creator : BusCreator  Inputs=3
  Constant13 : Constant  Value=RAND2  VectorParams1D=off  SampleTime=ts_opti
  Data Store Read : DataStoreRead  DataStoreName=Y2  SampleTime=ts_opti  DataStoreElements=Y2
  Data Store Read1 : DataStoreRead  DataStoreName=X2  SampleTime=ts_opti  DataStoreElements=X2
  Demux : Demux
  MATLAB Function : MATLAB Function  TreatAsAtomicUnit=on
  MATLAB Function1 : MATLAB Function  TreatAsAtomicUnit=on
  Scope : Scope
  SIGMA : Outport
  sf : Outport  Port=2
  ell : Outport  Port=3
  wires:
  hyp_init/1 -> MATLAB Function/1(hyp_init)
  MATLAB Function/2(beta_out) -> Scope/1  "beta"
  Data Store Read1/1 -> MATLAB Function/2(x)
  Data Store Read/1 -> MATLAB Function/3(y)
  sn/1 -> MATLAB Function/4(sn2)
  Demux/4 -> sf/1  "sf"
  Constant13/1 -> MATLAB Function1/1(RAND)
  MATLAB Function1/1(SIGMA) -> SIGMA/1
  MATLAB Function/1(hyp_opt) -> Demux/1, MATLAB Function1/2(hyp)
  Demux/1 -> Bus Creator/1  "l_1"
  Demux/2 -> Bus Creator/2  "l_2"
  Demux/3 -> Bus Creator/3  "l_3"
  Bus Creator/1 -> ell/1

== system TFlex_ISSGP_Twin/TDfhan ==
  V : Inport
  P_init : Inport  Port=2
  Bus Creator : BusCreator  Inputs=3
  Constant : Constant  Value=Reference.transient.r  SampleTime=ts
  Constant1 : Constant  Value=Reference.transient.h  SampleTime=ts
  Discrete-Time Integrator : DiscreteIntegrator  gainval=1  SampleTime=ts  ICPrevOutput=DiscIntNeverNeededParam  ICPrevScaledInput=DiscIntNeverNeededParam
  Discrete-Time Integrator1 : DiscreteIntegrator  gainval=1  InitialConditionSource=external  InitialCondition=-24  SampleTime=ts  ICPrevOutput=DiscIntNeverNeededParam  ICPrevScaledInput=DiscIntNeverNeededParam
  MATLAB Function2 : MATLAB Function  TreatAsAtomicUnit=on
  Scope : Scope  NumInputPorts=3
  Sum : Sum  Inputs=+-|
  ref : Outport
  wires:
  Sum/1 -> MATLAB Function2/1(v1)
  V/1 -> Sum/2
  Constant/1 -> MATLAB Function2/3(r0)
  Constant1/1 -> MATLAB Function2/4(h0)
  P_init/1 -> Discrete-Time Integrator1/2
  Discrete-Time Integrator1/1 -> Sum/1, Scope/1, Bus Creator/1  "r"
  Discrete-Time Integrator/1 -> Discrete-Time Integrator1/1, Scope/2, Bus Creator/2, MATLAB Function2/2(v2)  "r_dot"
  Bus Creator/1 -> ref/1
  MATLAB Function2/1(output) -> Scope/3, Bus Creator/3, Discrete-Time Integrator/1  "r_ddot"

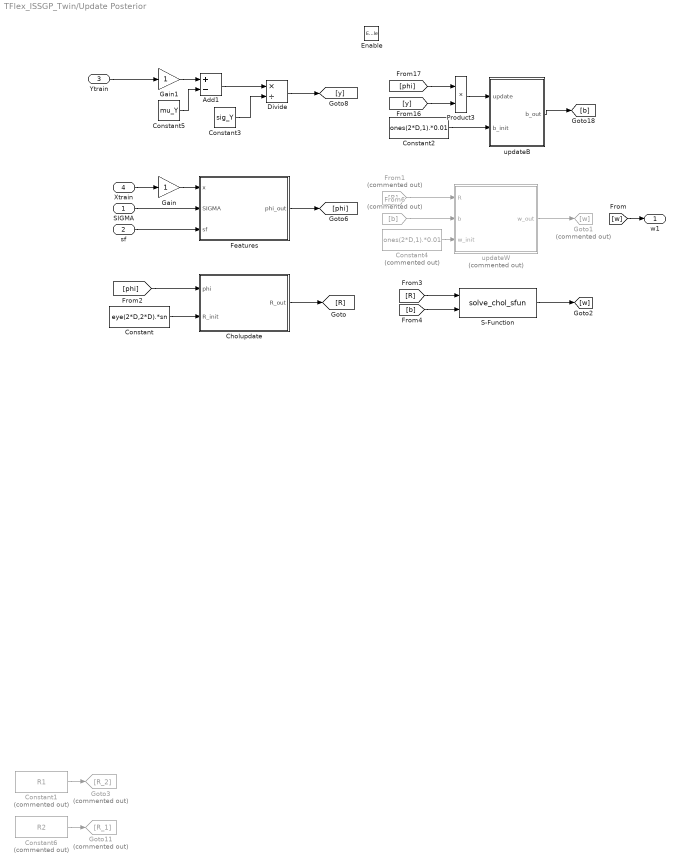
== system TFlex_ISSGP_Twin/Update Posterior ==
  SIGMA : Inport  SampleTime=ts
  sf : Inport  Port=2  SampleTime=ts
  Ytrain : Inport  Port=3  PortDimensions=[1,1]  SampleTime=ts
  Xtrain : Inport  Port=4  PortDimensions=[n,1]  SampleTime=ts
  Enable : EnablePort
  Add1 : Sum  Inputs=+-
  Cholupdate : MATLAB Function  TreatAsAtomicUnit=on
  Constant : Constant  Value=eye(2*D,2*D).*sn  SampleTime=ts
  Constant1 : Constant  Commented=on  Value=R1  VectorParams1D=off  SampleTime=-1
  Constant2 : Constant  Value=ones(2*D,1).*0.01  SampleTime=ts
  Constant3 : Constant  Value=sig_Y  VectorParams1D=off  SampleTime=ts
  Constant4 : Constant  Commented=on  Value=ones(2*D,1).*0.01  SampleTime=ts
  Constant5 : Constant  Value=mu_Y  VectorParams1D=off  SampleTime=ts
  Constant6 : Constant  Commented=on  Value=R2  VectorParams1D=off  SampleTime=-1
  Divide : Product  Inputs=*/
  Features : Subsystem
  From1 : From  Commented=on  GotoTag=R
  From6 : From  Commented=on  GotoTag=b
  Gain : Gain
  Gain1 : Gain
  Goto1 : Goto  Commented=on  GotoTag=w
  Goto11 : Goto  Commented=on  GotoTag=R_1
  Goto3 : Goto  Commented=on  GotoTag=R_2
  Product3 : Product
  S-Function : S-Function  FunctionName=solve_chol_sfun  Parameters=2*D  SFunctionDeploymentMode=off  EnableBusSupport=off
  updateB : MATLAB Function  TreatAsAtomicUnit=on
  updateW : MATLAB Function  Commented=on  TreatAsAtomicUnit=on
  w1 : Outport
  wires:
  Divide/1 -> [y]
  [phi] -> Cholupdate/1(phi)
  Features/1(phi_out) -> [phi]
  Cholupdate/1(R_out) -> [R]
  Constant3/1 -> Divide/2
  Constant5/1 -> Add1/2
  Add1/1 -> Divide/1
  From1/1 -> updateW/1(R)
  From6/1 -> updateW/2(b)
  Constant1/1 -> Goto3/1
  Constant6/1 -> Goto11/1
  [y] -> Product3/2
  [phi] -> Product3/1
  Product3/1 -> updateB/1(update)
  updateB/1(b_out) -> [b]
  SIGMA/1 -> Features/2(SIGMA)
  sf/1 -> Features/3(sf)
  Gain/1 -> Features/1(x)
  Gain1/1 -> Add1/1
  Constant/1 -> Cholupdate/2(R_init)
  Constant2/1 -> updateB/2(b_init)
  Constant4/1 -> updateW/3(w_init)
  Ytrain/1 -> Gain1/1
  Xtrain/1 -> Gain/1
  [R] -> S-Function/1
  [b] -> S-Function/2
  [w] -> w1/1
  updateW/1(w_out) -> Goto1/1
  S-Function/1 -> [w]

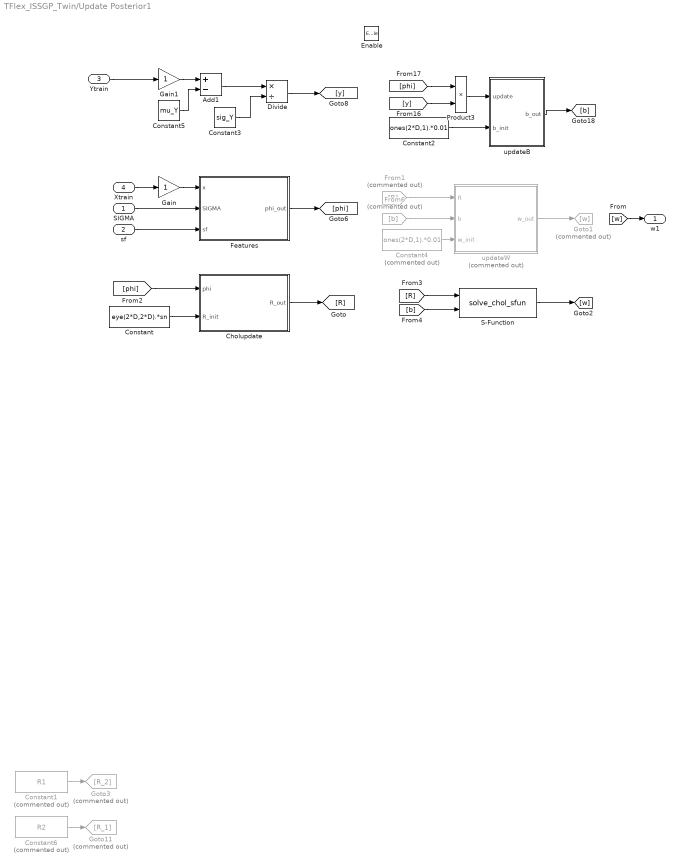
== system TFlex_ISSGP_Twin/Update Posterior1 ==
  SIGMA : Inport  SampleTime=ts
  sf : Inport  Port=2  SampleTime=ts
  Ytrain : Inport  Port=3  PortDimensions=[1,1]  SampleTime=ts
  Xtrain : Inport  Port=4  PortDimensions=[n,1]  SampleTime=ts
  Enable : EnablePort
  Add1 : Sum  Inputs=+-
  Cholupdate : MATLAB Function  TreatAsAtomicUnit=on
  Constant : Constant  Value=eye(2*D,2*D).*sn  SampleTime=ts
  Constant1 : Constant  Commented=on  Value=R1  VectorParams1D=off  SampleTime=-1
  Constant2 : Constant  Value=ones(2*D,1).*0.01  SampleTime=ts
  Constant3 : Constant  Value=sig_Y  VectorParams1D=off  SampleTime=ts
  Constant4 : Constant  Commented=on  Value=ones(2*D,1).*0.01  SampleTime=ts
  Constant5 : Constant  Value=mu_Y  VectorParams1D=off  SampleTime=ts
  Constant6 : Constant  Commented=on  Value=R2  VectorParams1D=off  SampleTime=-1
  Divide : Product  Inputs=*/
  Features : Subsystem
  From1 : From  Commented=on  GotoTag=R
  From6 : From  Commented=on  GotoTag=b
  Gain : Gain
  Gain1 : Gain
  Goto1 : Goto  Commented=on  GotoTag=w
  Goto11 : Goto  Commented=on  GotoTag=R_1
  Goto3 : Goto  Commented=on  GotoTag=R_2
  Product3 : Product
  S-Function : S-Function  FunctionName=solve_chol_sfun  Parameters=2*D  SFunctionDeploymentMode=off  EnableBusSupport=off
  updateB : MATLAB Function  TreatAsAtomicUnit=on
  updateW : MATLAB Function  Commented=on  TreatAsAtomicUnit=on
  w1 : Outport
  wires:
  Divide/1 -> [y]
  [phi] -> Cholupdate/1(phi)
  Features/1(phi_out) -> [phi]
  Cholupdate/1(R_out) -> [R]
  Constant3/1 -> Divide/2
  Constant5/1 -> Add1/2
  Add1/1 -> Divide/1
  From1/1 -> updateW/1(R)
  From6/1 -> updateW/2(b)
  Constant1/1 -> Goto3/1
  Constant6/1 -> Goto11/1
  [y] -> Product3/2
  [phi] -> Product3/1
  Product3/1 -> updateB/1(update)
  updateB/1(b_out) -> [b]
  SIGMA/1 -> Features/2(SIGMA)
  sf/1 -> Features/3(sf)
  Gain/1 -> Features/1(x)
  Gain1/1 -> Add1/1
  Constant/1 -> Cholupdate/2(R_init)
  Constant2/1 -> updateB/2(b_init)
  Constant4/1 -> updateW/3(w_init)
  Ytrain/1 -> Gain1/1
  Xtrain/1 -> Gain/1
  [R] -> S-Function/1
  [b] -> S-Function/2
  [w] -> w1/1
  updateW/1(w_out) -> Goto1/1
  S-Function/1 -> [w]

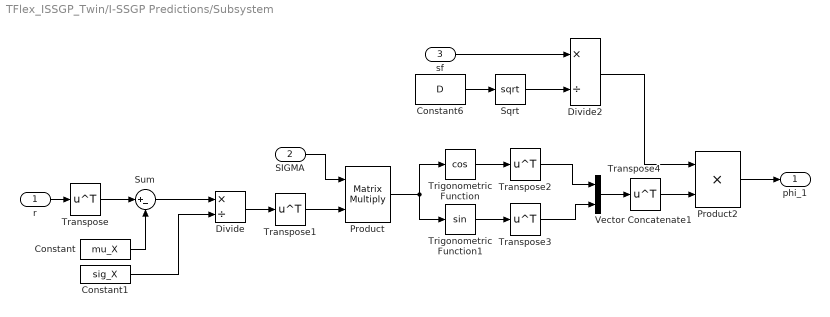
== system TFlex_ISSGP_Twin/I-SSGP Predictions/Subsystem ==
  r : Inport
  SIGMA : Inport  Port=2
  sf : Inport  Port=3
  Constant : Constant  Value=mu_X  VectorParams1D=off  SampleTime=-1
  Constant1 : Constant  Value=sig_X  VectorParams1D=off  SampleTime=-1
  Constant6 : Constant  Value=D  SampleTime=-1
  Divide : Product  Inputs=*/
  Divide2 : Product  Inputs=*/
  Product : Product  Multiplication=Matrix(*)
  Product2 : Product
  Sqrt : Sqrt  SaturateOnIntegerOverflow=on
  Sum : Sum  Inputs=|+-
  Transpose{,1..4} (5 alike) : Math  Operator=transpose  SaturateOnIntegerOverflow=on
  Trigonometric Function : Trigonometry  Operator=cos
  Trigonometric Function1 : Trigonometry
  Vector Concatenate1 : Concatenate
  phi_1 : Outport
  wires:
  Transpose1/1 -> Product/2
  Divide/1 -> Transpose1/1
  r/1 -> Transpose/1
  Product/1 -> Trigonometric Function1/1, Trigonometric Function/1
  Product2/1 -> phi_1/1
  sf/1 -> Divide2/1
  Divide2/1 -> Product2/1
  Sum/1 -> Divide/1
  Constant1/1 -> Divide/2
  Constant/1 -> Sum/2
  Transpose2/1 -> Vector Concatenate1/1
  Transpose4/1 -> Product2/2
  Constant6/1 -> Sqrt/1
  Trigonometric Function1/1 -> Transpose3/1
  Trigonometric Function/1 -> Transpose2/1
  Vector Concatenate1/1 -> Transpose4/1
  Transpose3/1 -> Vector Concatenate1/2
  Sqrt/1 -> Divide2/2
  SIGMA/1 -> Product/1
  Transpose/1 -> Sum/1

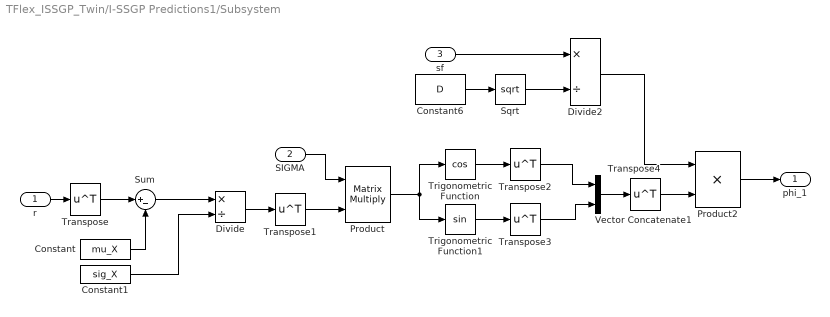
== system TFlex_ISSGP_Twin/I-SSGP Predictions1/Subsystem ==
  r : Inport
  SIGMA : Inport  Port=2
  sf : Inport  Port=3
  Constant : Constant  Value=mu_X  VectorParams1D=off  SampleTime=-1
  Constant1 : Constant  Value=sig_X  VectorParams1D=off  SampleTime=-1
  Constant6 : Constant  Value=D  SampleTime=-1
  Divide : Product  Inputs=*/
  Divide2 : Product  Inputs=*/
  Product : Product  Multiplication=Matrix(*)
  Product2 : Product
  Sqrt : Sqrt  SaturateOnIntegerOverflow=on
  Sum : Sum  Inputs=|+-
  Transpose{,1..4} (5 alike) : Math  Operator=transpose  SaturateOnIntegerOverflow=on
  Trigonometric Function : Trigonometry  Operator=cos
  Trigonometric Function1 : Trigonometry
  Vector Concatenate1 : Concatenate
  phi_1 : Outport
  wires:
  Transpose1/1 -> Product/2
  Divide/1 -> Transpose1/1
  r/1 -> Transpose/1
  Product/1 -> Trigonometric Function1/1, Trigonometric Function/1
  Product2/1 -> phi_1/1
  sf/1 -> Divide2/1
  Divide2/1 -> Product2/1
  Sum/1 -> Divide/1
  Constant1/1 -> Divide/2
  Constant/1 -> Sum/2
  Transpose2/1 -> Vector Concatenate1/1
  Transpose4/1 -> Product2/2
  Constant6/1 -> Sqrt/1
  Trigonometric Function1/1 -> Transpose3/1
  Trigonometric Function/1 -> Transpose2/1
  Vector Concatenate1/1 -> Transpose4/1
  Transpose3/1 -> Vector Concatenate1/2
  Sqrt/1 -> Divide2/2
  SIGMA/1 -> Product/1
  Transpose/1 -> Sum/1

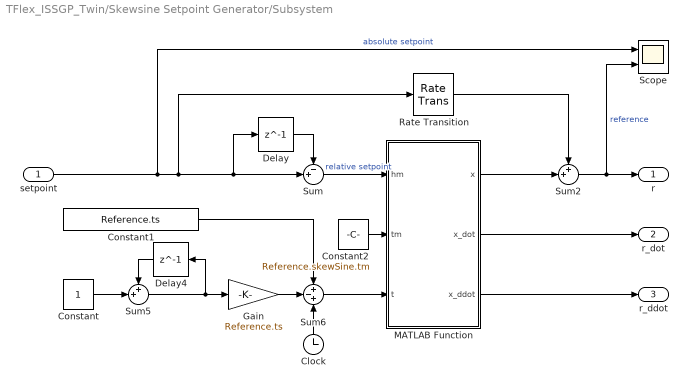
== system TFlex_ISSGP_Twin/Skewsine Setpoint Generator/Subsystem ==
  setpoint : Inport
  Clock : Clock
      settings: Decimation=100
  Constant : Constant  SampleTime=Reference.ts
  Constant1 : Constant  Value=Reference.ts  SampleTime=Reference.ts
  Constant2 : Constant  Value=Reference.skewSine.tm  SampleTime=Reference.ts
  Delay : Delay  DelayLength=1  InitialCondition=0  SampleTime=Reference.ts
  Delay4 : Delay  DelayLength=1  InitialCondition=0  SampleTime=Reference.ts
  Gain : Gain  Gain=Reference.ts
  MATLAB Function : MATLAB Function  TreatAsAtomicUnit=on
  Rate Transition : RateTransition  OutPortSampleTime=ts
  Scope : Scope  NumInputPorts=2
  Sum : Sum  Inputs=-+|
  Sum2 : Sum  Inputs=++|
  Sum5 : Sum  Inputs=++|
  Sum6 : Sum  Inputs=+-+
  r : Outport
  r_dot : Outport  Port=2
  r_ddot : Outport  Port=3
  wires:
  Delay4/1 -> Sum5/1
  Sum2/1 -> r/1, Scope/2  "reference"
  Sum5/1 -> Delay4/1, Gain/1
  Constant/1 -> Sum5/2
  MATLAB Function/3(x_ddot) -> r_ddot/1
  Clock/1 -> Sum6/3
  Delay/1 -> Sum/1
  Gain/1 -> Sum6/2
  Constant1/1 -> Sum6/1
  MATLAB Function/2(x_dot) -> r_dot/1
  Sum/1 -> MATLAB Function/1(hm)  "relative setpoint"
  Constant2/1 -> MATLAB Function/2(tm)
  Sum6/1 -> MATLAB Function/3(t)
  MATLAB Function/1(x) -> Sum2/2
  setpoint/1 -> Scope/1, Rate Transition/1, Delay/1, Sum/2  "absolute setpoint"
  Rate Transition/1 -> Sum2/1

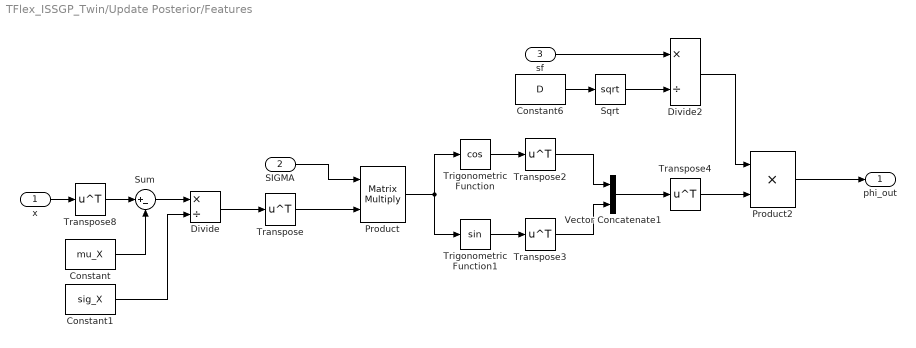
== system TFlex_ISSGP_Twin/Update Posterior/Features ==
  x : Inport
  SIGMA : Inport  Port=2
  sf : Inport  Port=3
  Constant : Constant  Value=mu_X  VectorParams1D=off  SampleTime=ts
  Constant1 : Constant  Value=sig_X  VectorParams1D=off  SampleTime=ts
  Constant6 : Constant  Value=D  SampleTime=-1
  Divide : Product  Inputs=*/
  Divide2 : Product  Inputs=*/
  Product : Product  Multiplication=Matrix(*)
  Product2 : Product
  Sqrt : Sqrt  SaturateOnIntegerOverflow=on
  Sum : Sum  Inputs=|+-
  Transpose{,2..4,8} (5 alike) : Math  Operator=transpose  SaturateOnIntegerOverflow=on
  Trigonometric Function : Trigonometry  Operator=cos
  Trigonometric Function1 : Trigonometry
  Vector Concatenate1 : Concatenate
  phi_out : Outport
  wires:
  Sum/1 -> Divide/1
  SIGMA/1 -> Product/1
  Product2/1 -> phi_out/1
  Constant6/1 -> Sqrt/1
  Trigonometric Function1/1 -> Transpose3/1
  Trigonometric Function/1 -> Transpose2/1
  Vector Concatenate1/1 -> Transpose4/1
  Transpose3/1 -> Vector Concatenate1/2
  Product/1 -> Trigonometric Function1/1, Trigonometric Function/1
  Constant1/1 -> Divide/2
  Transpose/1 -> Product/2
  Divide/1 -> Transpose/1
  Divide2/1 -> Product2/1
  Transpose4/1 -> Product2/2
  Sqrt/1 -> Divide2/2
  Constant/1 -> Sum/2
  Transpose2/1 -> Vector Concatenate1/1
  x/1 -> Transpose8/1
  Transpose8/1 -> Sum/1
  sf/1 -> Divide2/1

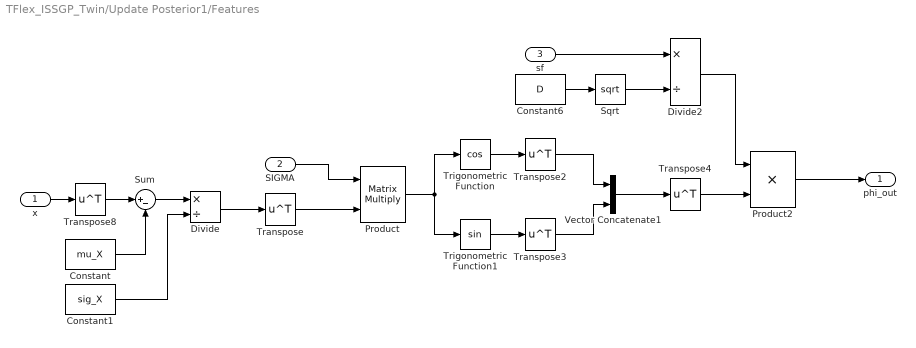
== system TFlex_ISSGP_Twin/Update Posterior1/Features ==
  x : Inport
  SIGMA : Inport  Port=2
  sf : Inport  Port=3
  Constant : Constant  Value=mu_X  VectorParams1D=off  SampleTime=ts
  Constant1 : Constant  Value=sig_X  VectorParams1D=off  SampleTime=ts
  Constant6 : Constant  Value=D  SampleTime=-1
  Divide : Product  Inputs=*/
  Divide2 : Product  Inputs=*/
  Product : Product  Multiplication=Matrix(*)
  Product2 : Product
  Sqrt : Sqrt  SaturateOnIntegerOverflow=on
  Sum : Sum  Inputs=|+-
  Transpose{,2..4,8} (5 alike) : Math  Operator=transpose  SaturateOnIntegerOverflow=on
  Trigonometric Function : Trigonometry  Operator=cos
  Trigonometric Function1 : Trigonometry
  Vector Concatenate1 : Concatenate
  phi_out : Outport
  wires:
  Sum/1 -> Divide/1
  SIGMA/1 -> Product/1
  Product2/1 -> phi_out/1
  Constant6/1 -> Sqrt/1
  Trigonometric Function1/1 -> Transpose3/1
  Trigonometric Function/1 -> Transpose2/1
  Vector Concatenate1/1 -> Transpose4/1
  Transpose3/1 -> Vector Concatenate1/2
  Product/1 -> Trigonometric Function1/1, Trigonometric Function/1
  Constant1/1 -> Divide/2
  Transpose/1 -> Product/2
  Divide/1 -> Transpose/1
  Divide2/1 -> Product2/1
  Transpose4/1 -> Product2/2
  Sqrt/1 -> Divide2/2
  Constant/1 -> Sum/2
  Transpose2/1 -> Vector Concatenate1/1
  x/1 -> Transpose8/1
  Transpose8/1 -> Sum/1
  sf/1 -> Divide2/1

== matlab function TFlex_ISSGP_Twin/Subsystem1/MATLAB Function2 ==
  data: x input; X data_store_memory
function writeTo(x)
global X
X = [X(2:end,:);x];

== matlab function TFlex_ISSGP_Twin/Skewsine Setpoint Generator/Subsystem/MATLAB Function ==
  settings: updateMethod=DISCRETE  sampleTime=ts
  data: hm input; x output; tm input; t input; x_dot output; x_ddot output
function [x,x_dot,x_ddot] = skewSine(hm,tm,t)

if (t>=0) && (t<=tm)
    x      = hm/tm*t - hm/(2*pi)*sin(2*pi/tm*t);
    x_dot  = hm/tm - hm/tm*cos(2*pi/tm*t);
    x_ddot = 2*pi*hm/(tm^2)*sin(2*pi/tm*t);
else
    x      = hm;
    x_dot  = 0;
    x_ddot = 0;
end

== matlab function TFlex_ISSGP_Twin/Subsystem/MATLAB Function1 ==
  data: RAND input; SIGMA output; hyp input
function SIGMA  = fcn(RAND,hyp)

SIGMA = zeros(size(RAND));
SIGMA(:,1) = RAND(:,1).*hyp(1);
SIGMA(:,2) = RAND(:,2).*hyp(2);
SIGMA(:,3) = RAND(:,3).*hyp(3);

== matlab function TFlex_ISSGP_Twin/Update Posterior/updateW ==
  settings: updateMethod=DISCRETE  sampleTime=ts
  data: R input size=[2*D,2*D]; w_out output size=[2*D,1]; b input; w_init input; D parameter
function w_out = updateW(R,b,w_init,D) 
persistent w
if(isempty(w))
    w = w_init;
end
coder.extrinsic('solve_chol');
w = solve_chol(R,b);
%w = R\(R'\b);
w_out = w;

== matlab function TFlex_ISSGP_Twin/Subsystem2/MATLAB Function ==
  data: Vr input; y output; p input
function y = fcn(Vr,p)
if Vr>0 && p>=17
    y = Vr;
elseif Vr<0 && p<=-17
    y = Vr;
else
    y = 0;
end

== matlab function TFlex_ISSGP_Twin/Update Posterior/Cholupdate ==
  settings: updateMethod=DISCRETE  sampleTime=ts
  data: R_out output size=[2*D,2*D]; phi input; R_init input; D parameter; sn parameter
function R_out = cholupdate_fcn(phi, R_init, D, sn)
persistent R; 
if(isempty(R))
    R = R_init;
end
R = cholupdate(R,phi);
R_out = R;

== matlab function TFlex_ISSGP_Twin/TDfhan/MATLAB Function2 ==
  data: v1 input; output output; v2 input; r0 input; h0 input
function output = Fhan(v1,v2,r0, h0)
d = h0^2*r0;
a0 = h0*v2;
y = v1 + a0;
a1 = sqrt(d*(d+8*abs(y)));
a2 = a0 + sign(y)*(a1-d)/2;
sy = (sign(y+d)-sign(y-d))/2;
a = (a0+y-a2)*sy +a2;
sa = (sign(a+d)-sign(a-d))/2;
output = -r0 *(a/d -sign(a) )*sa - r0*sign(a);

== matlab function TFlex_ISSGP_Twin/Update Posterior/updateB ==
  settings: updateMethod=DISCRETE  sampleTime=ts
  data: update input; b_init input; b_out output size=[2*D,1]; D parameter
function b_out = updateB(update, b_init, D)
persistent b 
if(isempty(b))
    b = b_init;
end

b = b + update;
b_out = b;

== matlab function TFlex_ISSGP_Twin/Update Posterior1/Cholupdate ==
  settings: updateMethod=DISCRETE  sampleTime=ts
  data: R_out output size=[2*D,2*D]; phi input; R_init input; D parameter; sn parameter
function R_out = cholupdate_fcn(phi, R_init, D, sn)
persistent R; 
if(isempty(R))
    R = R_init;
end
R = cholupdate(R,phi);
R_out = R;

== matlab function TFlex_ISSGP_Twin/Update Posterior1/updateB ==
  settings: updateMethod=DISCRETE  sampleTime=ts
  data: update input; b_init input; b_out output size=[2*D,1]; D parameter
function b_out = updateB(update, b_init, D)
persistent b 
if(isempty(b))
    b = b_init;
end

b = b + update;
b_out = b;

== matlab function TFlex_ISSGP_Twin/Update Posterior1/updateW ==
  settings: updateMethod=DISCRETE  sampleTime=ts
  data: R input size=[2*D,2*D]; w_out output size=[2*D,1]; b input; w_init input; D parameter
function w_out = updateW(R,b,w_init,D) 
persistent w
if(isempty(w))
    w = w_init;
end
coder.extrinsic('solve_chol');
w = solve_chol(R,b);
%w = R\(R'\b);
w_out = w;

== matlab function TFlex_ISSGP_Twin/Subsystem3/MATLAB Function1 ==
  data: y input; Y2 data_store_memory
function writeTo(y)
global Y2

Y2 = [Y2(2:end,:);y'];

== matlab function TFlex_ISSGP_Twin/Subsystem3/MATLAB Function2 ==
  data: x input; X2 data_store_memory
function writeTo(x)
global X2

X2 = [X2(2:end,:);x];

== matlab function TFlex_ISSGP_Twin/Subsystem/MATLAB Function ==
  data: hyp_init input; hyp_opt output; x input; y input; Z parameter; D parameter; RAND parameter; n parameter; sn2 input; beta_out output; beta_init parameter; beta_min parameter; beta_reduc parameter
function [hyp_opt,beta_out]= hyperparamUpdate(hyp_init,x,y,Z,D,RAND,n,sn2,beta_init, beta_min, beta_reduc)
coder.extrinsic('opt_hyperparam');
persistent hyp1 beta
if(isempty(hyp1))
    hyp1 = hyp_init;
    beta = beta_init;
end
hyp_opt = hyp1;
hyp_new = zeros(size(hyp_init));

hyp_new = opt_hyperparam(hyp_opt,x,y,sn2,Z,D,RAND,n);
hyp1 = hyp_opt.*(1-beta) + beta.*hyp_new;
hyp_opt = hyp1;


beta_new = beta.*beta_reduc;
beta = max(beta_new,beta_min);
beta_out = beta;

== matlab function TFlex_ISSGP_Twin/Subsystem1/MATLAB Function1 ==
  data: y input; Y data_store_memory
function writeTo(y)
global Y

Y = [Y(2:end,:);y'];

== matlab function TFlex_ISSGP_Twin/Subsystem4/MATLAB Function ==
  data: hyp_init input; hyp_opt output; x input; y input; Z parameter; D parameter; RAND parameter; n parameter; sn2 input; beta_out output; beta_init parameter; beta_min parameter; beta_reduc parameter
function [hyp_opt,beta_out]= hyperparamUpdate(hyp_init,x,y,Z,D,RAND,n,sn2,beta_init, beta_min, beta_reduc)
coder.extrinsic('opt_hyperparam');
persistent hyp1 beta
if(isempty(hyp1))
    hyp1 = hyp_init;
    beta = beta_init;
end
hyp_opt = hyp1;
hyp_new = zeros(size(hyp_init));

hyp_new = opt_hyperparam(hyp_opt,x,y,sn2,Z,D,RAND,n);
hyp1 = hyp_opt.*(1-beta) + beta.*hyp_new;
hyp_opt = hyp1;


beta_new = beta.*beta_reduc;
beta = max(beta_new,beta_min);
beta_out = beta;

== matlab function TFlex_ISSGP_Twin/Subsystem4/MATLAB Function1 ==
  data: RAND input; SIGMA output; hyp input
function SIGMA  = fcn(RAND,hyp)

SIGMA = zeros(size(RAND));
SIGMA(:,1) = RAND(:,1).*hyp(1);
SIGMA(:,2) = RAND(:,2).*hyp(2);
SIGMA(:,3) = RAND(:,3).*hyp(3);
